simulink model "pump_v000"  (R2019b)
settings: Solver=ode4  StartTime=0.0  StopTime=100  FixedStep=0.02  RelTol=1e-3
libraries: simulink x6
settings Model: PauseTimes=11.82  Creator=engineer  LastModifiedBy=engineer

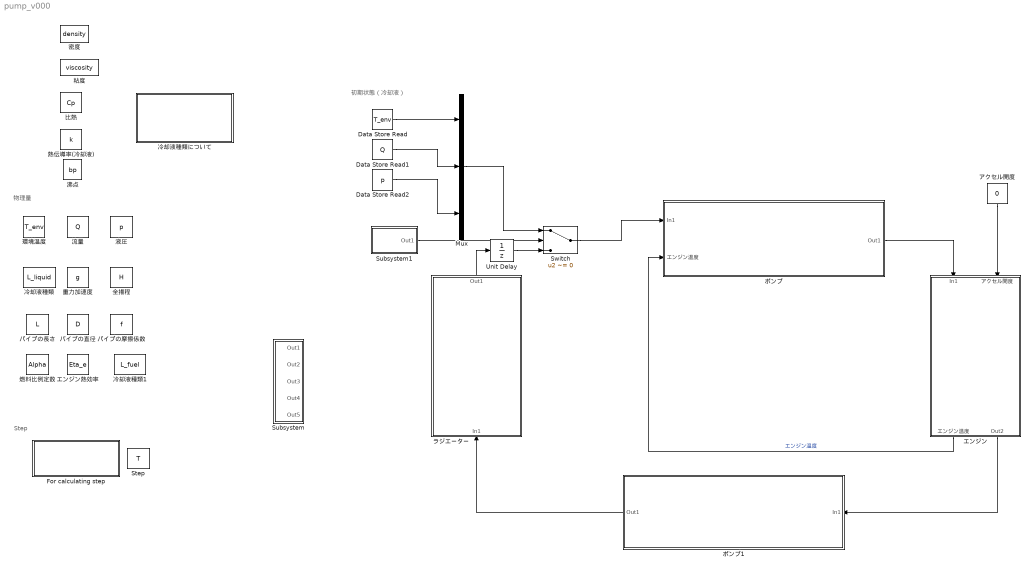
== system pump_v000 ==
  note: 初期状態（冷却液）
  note: 物理量
  note: Step
  " 全揚程" : DataStoreMemory  DataStoreName=H  ReadBeforeWriteMsg=warning  WriteAfterWriteMsg=warning  WriteAfterReadMsg=warning  InitialValue=2  ShowAdditionalParam=off
  " 冷却液種類" : DataStoreMemory  DataStoreName=L_liquid  ReadBeforeWriteMsg=warning  WriteAfterWriteMsg=warning  WriteAfterReadMsg=warning  ShowAdditionalParam=off  OutMin=0  OutMax=2
  " 冷却液種類1" : DataStoreMemory  DataStoreName=L_fuel  ReadBeforeWriteMsg=warning  WriteAfterWriteMsg=warning  WriteAfterReadMsg=warning  ShowAdditionalParam=off  OutMin=0  OutMax=2
  " 流量" : DataStoreMemory  DataStoreName=Q  ReadBeforeWriteMsg=warning  WriteAfterWriteMsg=warning  WriteAfterReadMsg=warning  ShowAdditionalParam=off
  " 液圧" : DataStoreMemory  DataStoreName=p  ReadBeforeWriteMsg=warning  WriteAfterWriteMsg=warning  WriteAfterReadMsg=warning  InitialValue=1  ShowAdditionalParam=off
  " 重力加速度" : DataStoreMemory  DataStoreName=g  ReadBeforeWriteMsg=warning  WriteAfterWriteMsg=warning  WriteAfterReadMsg=warning  InitialValue=10  ShowAdditionalParam=off
  Data Store Read : DataStoreRead  DataStoreName=T_env
  Data Store Read1 : DataStoreRead  DataStoreName=Q
  Data Store Read2 : DataStoreRead  DataStoreName=p
  For calculating step : Subsystem
  Mux : Mux  Inputs=3
  Step : DataStoreMemory  DataStoreName=T  ReadBeforeWriteMsg=warning  WriteAfterWriteMsg=warning  WriteAfterReadMsg=warning  ShowAdditionalParam=off
  Subsystem : Subsystem
  Subsystem1 : Subsystem
  Switch : Switch  Criteria=u2 ~= 0
  Unit Delay : UnitDelay  SampleTime=-1  HasFrameUpgradeWarning=on
  アクセル開度 : Constant  Value=0
  エンジン : Subsystem
  エンジン熱効率 : DataStoreMemory  DataStoreName=Eta_e  ReadBeforeWriteMsg=warning  WriteAfterWriteMsg=warning  WriteAfterReadMsg=warning  InitialValue=0.1  ShowAdditionalParam=off
  パイプの摩擦係数 : DataStoreMemory  DataStoreName=f  ReadBeforeWriteMsg=warning  WriteAfterWriteMsg=warning  WriteAfterReadMsg=warning  InitialValue=0.01  ShowAdditionalParam=off
  パイプの直径 : DataStoreMemory  DataStoreName=D  ReadBeforeWriteMsg=warning  WriteAfterWriteMsg=warning  WriteAfterReadMsg=warning  InitialValue=0.04  ShowAdditionalParam=off
  パイプの長さ : DataStoreMemory  DataStoreName=L  ReadBeforeWriteMsg=warning  WriteAfterWriteMsg=warning  WriteAfterReadMsg=warning  InitialValue=7  ShowAdditionalParam=off
  ポンプ : Subsystem
  ポンプ1 : Subsystem
  ラジエーター : Subsystem
  冷却液種類について : Subsystem
  密度 : DataStoreMemory  DataStoreName=density  ReadBeforeWriteMsg=warning  WriteAfterWriteMsg=warning  WriteAfterReadMsg=warning  ShowAdditionalParam=off
  比熱 : DataStoreMemory  DataStoreName=Cp  ReadBeforeWriteMsg=warning  WriteAfterWriteMsg=warning  WriteAfterReadMsg=warning  ShowAdditionalParam=off
  沸点 : DataStoreMemory  DataStoreName=bp  ReadBeforeWriteMsg=warning  WriteAfterWriteMsg=warning  WriteAfterReadMsg=warning  ShowAdditionalParam=off
  熱伝導率(冷却液) : DataStoreMemory  DataStoreName=k  ReadBeforeWriteMsg=warning  WriteAfterWriteMsg=warning  WriteAfterReadMsg=warning  ShowAdditionalParam=off
  燃料比例定数 : DataStoreMemory  DataStoreName=Alpha  ReadBeforeWriteMsg=warning  WriteAfterWriteMsg=warning  WriteAfterReadMsg=warning  InitialValue=0.005  ShowAdditionalParam=off
  "環境温度 " : DataStoreMemory  DataStoreName=T_env  ReadBeforeWriteMsg=warning  WriteAfterWriteMsg=warning  WriteAfterReadMsg=warning  InitialValue=25  ShowAdditionalParam=off
  粘度 : DataStoreMemory  DataStoreName=viscosity  ReadBeforeWriteMsg=warning  WriteAfterWriteMsg=warning  WriteAfterReadMsg=warning  ShowAdditionalParam=off
  wires:
  ポンプ/1(Out1) -> エンジン/1(In1)
  エンジン/2(Out2) -> ポンプ1/1(In1)
  ポンプ1/1(Out1) -> ラジエーター/1(In1)
  Mux/1 -> Switch/1
  Data Store Read/1 -> Mux/1
  Data Store Read1/1 -> Mux/2
  Data Store Read2/1 -> Mux/3
  Switch/1 -> ポンプ/1(In1)
  ラジエーター/1(Out1) -> Unit Delay/1
  Subsystem1/1(Out1) -> Switch/2
  エンジン/1(エンジン温度) -> ポンプ/2(エンジン温度)  "エンジン温度"
  Unit Delay/1 -> Switch/3
  アクセル開度/1 -> エンジン/2(アクセル開度)

== system pump_v000/For calculating step ==
  Add1 : Sum  Inputs=+-
  Clock1 : Clock
  Data Store Write : DataStoreWrite  DataStoreName=T
  Unit Delay2 : UnitDelay  SampleTime=-1  HasFrameUpgradeWarning=on
  wires:
  Clock1/1 -> Add1/1, Unit Delay2/1
  Add1/1 -> Data Store Write/1
  Unit Delay2/1 -> Add1/2

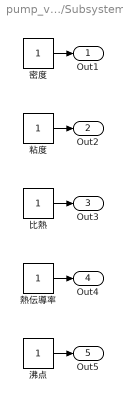
== system pump_v000/Subsystem ==
  密度 : Constant
  比熱 : Constant
  沸点 : Constant
  熱伝導率 : Constant
  粘度 : Constant
  Out1 : Outport
  Out2 : Outport  Port=2
  Out3 : Outport  Port=3
  Out4 : Outport  Port=4
  Out5 : Outport  Port=5
  wires:
  密度/1 -> Out1/1
  沸点/1 -> Out5/1
  比熱/1 -> Out3/1
  粘度/1 -> Out2/1
  熱伝導率/1 -> Out4/1

== system pump_v000/Subsystem1 ==
  Constant : Constant  OutDataTypeStr=boolean
  Logical Operator : Logic  Operator=NOT  AllPortsSameDT=off  OutDataTypeStr=boolean
  Logical Operator1 : Logic  AllPortsSameDT=off  OutDataTypeStr=boolean
  Unit Delay : UnitDelay  SampleTime=-1  HasFrameUpgradeWarning=on
  Out1 : Outport
  wires:
  Constant/1 -> Unit Delay/1, Logical Operator1/1
  Logical Operator/1 -> Logical Operator1/2
  Unit Delay/1 -> Logical Operator/1
  Logical Operator1/1 -> Out1/1

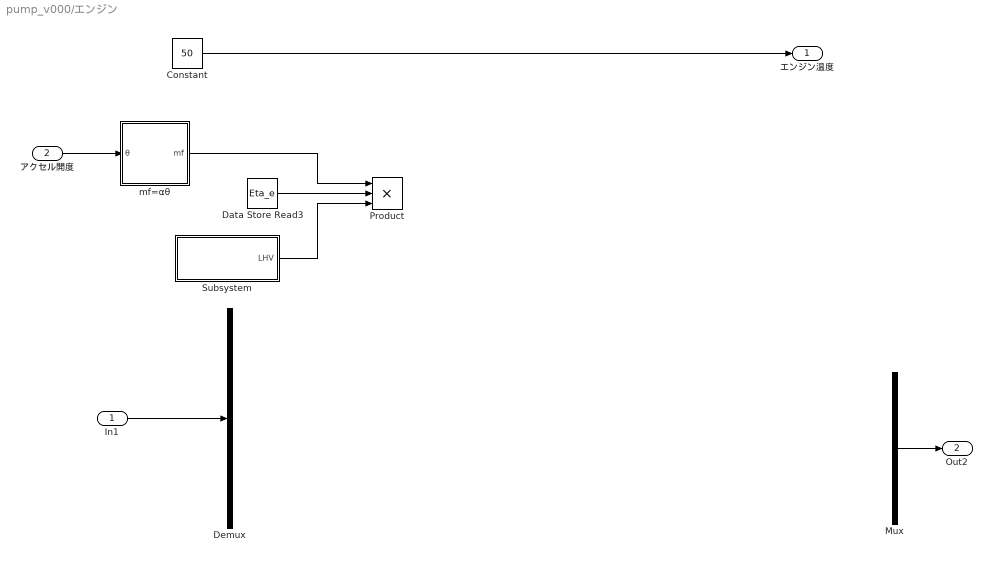
== system pump_v000/エンジン ==
  In1 : Inport
  アクセル開度 : Inport  Port=2
  Constant : Constant  Value=50
  Data Store Read3 : DataStoreRead  DataStoreName=Eta_e
  Demux : Demux  Outputs=3
  Mux : Mux  Inputs=3
  Product : Product  Inputs=3
  Subsystem : Subsystem
  mf=αθ : Subsystem
  エンジン温度 : Outport
  Out2 : Outport  Port=2
  wires:
  In1/1 -> Demux/1
  Constant/1 -> エンジン温度/1
  Mux/1 -> Out2/1
  アクセル開度/1 -> mf=αθ/1(θ)
  mf=αθ/1(mf) -> Product/1
  Data Store Read3/1 -> Product/2
  Subsystem/1("LHV ") -> Product/3

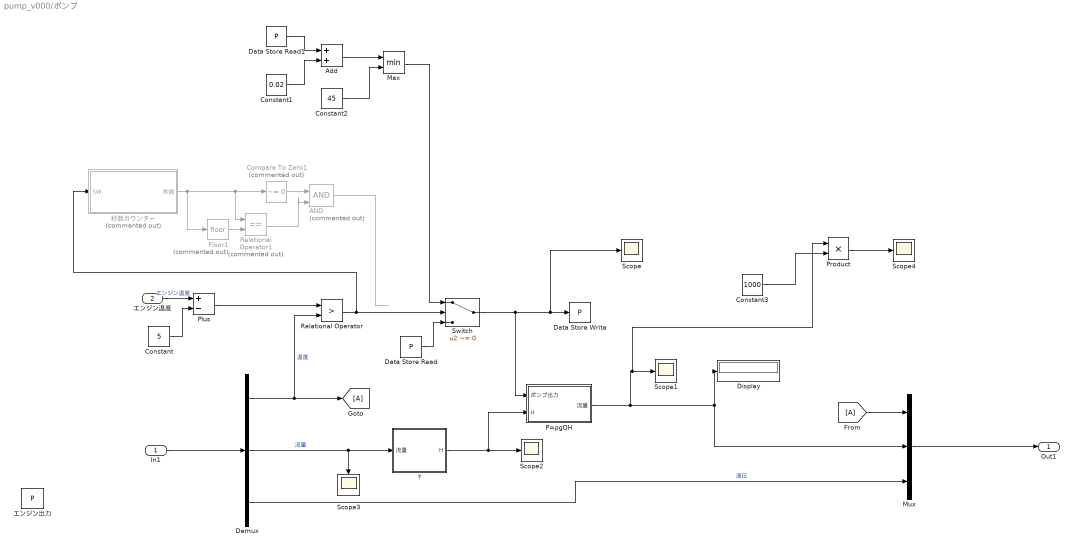
== system pump_v000/ポンプ ==
  In1 : Inport
  エンジン温度 : Inport  Port=2
  "?" : Subsystem
  AND : Logic  Commented=on  IconShape=distinctive  AllPortsSameDT=off  OutDataTypeStr=boolean
  Add : Sum
  Compare To Zero1 : simulink/Logic and Bit Operations/Compare To Zero  Commented=on  relop=~=  OutDataTypeStr=boolean
  Constant : Constant  Value=5
  Constant1 : Constant  Value=0.02
  Constant2 : Constant  Value=45
  Constant3 : Constant  Value=1000
  Data Store Read : DataStoreRead  DataStoreName=P
  Data Store Read1 : DataStoreRead  DataStoreName=P
  Data Store Write : DataStoreWrite  DataStoreName=P
  Demux : Demux  Outputs=3
  Display : Display
  Floor1 : Rounding  Commented=on
  Max : MinMax  Inputs=2
  Mux : Mux  Inputs=3
  P=ρgQH : Subsystem
  Plus : Sum  Inputs=+-
  Product : Product
  Relational Operator : RelationalOperator  Operator=>  OutDataTypeStr=boolean  RndMeth=Simplest
  Relational Operator1 : RelationalOperator  Commented=on  Operator===  OutDataTypeStr=boolean  RndMeth=Simplest
  Scope{,1..4} (5 alike) : Scope
  Switch : Switch  Criteria=u2 ~= 0
  エンジン出力 : DataStoreMemory  DataStoreName=P  ReadBeforeWriteMsg=warning  WriteAfterWriteMsg=warning  WriteAfterReadMsg=warning  ShowAdditionalParam=off
  秒数カウンター : Subsystem  Commented=on
  Out1 : Outport
  wires:
  In1/1 -> Demux/1
  Demux/3 -> Mux/3  "液圧"
  Demux/1 -> Relational Operator/2, [A]  "温度"
  P=ρgQH/1(流量) -> Display/1, Mux/2, Product/1, Scope1/1
  Constant/1 -> Plus/2
  エンジン温度/1 -> Plus/1  "エンジン温度"
  Plus/1 -> Relational Operator/1
  Switch/1 -> P=ρgQH/1(ポンプ出力), Scope/1, Data Store Write/1
  Data Store Read/1 -> Switch/3
  Data Store Read1/1 -> Add/1
  Constant1/1 -> Add/2
  Constant2/1 -> Max/2
  Add/1 -> Max/1
  Mux/1 -> Out1/1
  Demux/2 -> "?"/1(流量), Scope3/1  "流量"
  "?"/1(H) -> Scope2/1, P=ρgQH/2(H)
  [A] -> Mux/1
  Relational Operator1/1 -> AND/2
  秒数カウンター/1(秒数) -> Compare To Zero1/1, Relational Operator1/1, Floor1/1
  Floor1/1 -> Relational Operator1/2
  Compare To Zero1/1 -> AND/1
  AND/1 -> ?
  Max/1 -> Switch/1
  Relational Operator/1 -> Switch/2, 秒数カウンター/1(SW)
  Constant3/1 -> Product/2
  Product/1 -> Scope4/1

== system pump_v000/ポンプ1 ==
  In1 : Inport
  Out1 : Outport
  wires:
  In1/1 -> Out1/1

== system pump_v000/ラジエーター ==
  In1 : Inport
  Out1 : Outport
  wires:
  In1/1 -> Out1/1

== system pump_v000/冷却液種類について ==
  Compare To Constant : simulink/Logic and Bit Operations/Compare To Constant  relop===  const=0  OutDataTypeStr=boolean
  Compare To Constant1 : simulink/Logic and Bit Operations/Compare To Constant  relop===  const=1  OutDataTypeStr=boolean
  Compare To Constant2 : simulink/Logic and Bit Operations/Compare To Constant  relop===  const=2  OutDataTypeStr=boolean
  Data Store Read3 : DataStoreRead  DataStoreName=L_liquid
  Enabled Subsystem : Subsystem  TreatAsAtomicUnit=on
  Enabled Subsystem1 : Subsystem  TreatAsAtomicUnit=on
  Enabled Subsystem3 : Subsystem  TreatAsAtomicUnit=on
  wires:
  Compare To Constant/1 -> Enabled Subsystem/Enable  "水"
  Data Store Read3/1 -> Compare To Constant2/1, Compare To Constant1/1, Compare To Constant/1
  Compare To Constant1/1 -> Enabled Subsystem3/Enable  "EG(30%)"
  Compare To Constant2/1 -> Enabled Subsystem1/Enable  "EG(50%)"

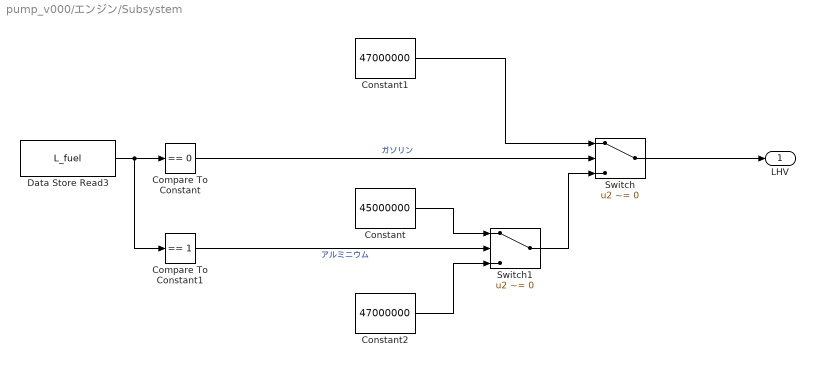
== system pump_v000/エンジン/Subsystem ==
  Compare To Constant : simulink/Logic and Bit Operations/Compare To Constant  relop===  const=0  OutDataTypeStr=boolean
  Compare To Constant1 : simulink/Logic and Bit Operations/Compare To Constant  relop===  const=1  OutDataTypeStr=boolean
  Constant : Constant  Value=45000000
  Constant1 : Constant  Value=47000000
  Constant2 : Constant  Value=47000000
  Data Store Read3 : DataStoreRead  DataStoreName=L_fuel
  Switch : Switch  Criteria=u2 ~= 0
  Switch1 : Switch  Criteria=u2 ~= 0
  "LHV " : Outport
  wires:
  Compare To Constant1/1 -> Switch1/2  "アルミニウム"
  Data Store Read3/1 -> Compare To Constant1/1, Compare To Constant/1
  Compare To Constant/1 -> Switch/2  "ガソリン"
  Switch/1 -> "LHV "/1
  Constant1/1 -> Switch/1
  Switch1/1 -> Switch/3
  Constant/1 -> Switch1/1
  Constant2/1 -> Switch1/3

== system pump_v000/エンジン/mf=αθ ==
  θ : Inport
  Constant1 : Constant  Value=0.02
  Data Store Read3 : DataStoreRead  DataStoreName=Alpha
  Product : Product  Inputs=3
  mf : Outport
  wires:
  Product/1 -> mf/1
  Data Store Read3/1 -> Product/2
  Constant1/1 -> Product/3
  θ/1 -> Product/1

== system pump_v000/ポンプ/? ==
  note: ?
  流量 : Inport
  Scope : Scope
  Scope1 : Scope
  hf=(fLv^2)/(2gD) : Subsystem
  v=Q/A : Subsystem
  ベルヌーイの定理 : Subsystem
  H : Outport
  wires:
  流量/1 -> Scope1/1, v=Q/A/1(Q)
  hf=(fLv^2)/(2gD)/1(hf) -> ベルヌーイの定理/1(hf)
  v=Q/A/1(v) -> ベルヌーイの定理/2(v), hf=(fLv^2)/(2gD)/1(v)
  ベルヌーイの定理/1(H) -> Scope/1, H/1

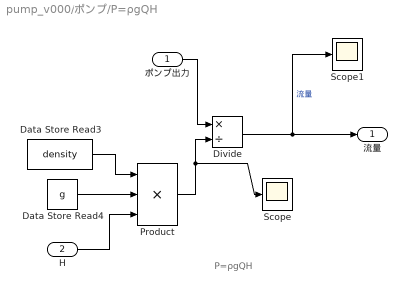
== system pump_v000/ポンプ/P=ρgQH ==
  note: P=ρgQH
  ポンプ出力 : Inport
  H : Inport  Port=2
  Data Store Read3 : DataStoreRead  DataStoreName=density
  Data Store Read4 : DataStoreRead  DataStoreName=g
  Divide : Product  Inputs=*/
  Product : Product  Inputs=3
  Scope : Scope
  Scope1 : Scope
  流量 : Outport
  wires:
  H/1 -> Product/3
  Data Store Read3/1 -> Product/1
  ポンプ出力/1 -> Divide/1
  Data Store Read4/1 -> Product/2
  Product/1 -> Scope/1, Divide/2
  Divide/1 -> Scope1/1, 流量/1  "流量"

== system pump_v000/ポンプ/秒数カウンター ==
  SW : Inport
  Add : Sum
  Constant1 : Constant  Value=0
  Data Store Read : DataStoreRead  DataStoreName=T
  Switch2 : Switch  Criteria=u2 ~= 0
  Unit Delay1 : UnitDelay  SampleTime=-1  HasFrameUpgradeWarning=on
  秒数 : Outport
  wires:
  SW/1 -> Switch2/2
  Add/1 -> Switch2/1
  Data Store Read/1 -> Add/2
  Constant1/1 -> Switch2/3
  Switch2/1 -> 秒数/1, Unit Delay1/1
  Unit Delay1/1 -> Add/1

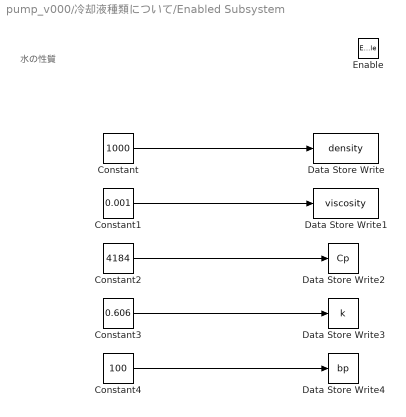
== system pump_v000/冷却液種類について/Enabled Subsystem ==
  note: 水の性質
  Enable : EnablePort
  Constant : Constant  Value=1000
  Constant1 : Constant  Value=0.001
  Constant2 : Constant  Value=4184
  Constant3 : Constant  Value=0.606
  Constant4 : Constant  Value=100
  Data Store Write : DataStoreWrite  DataStoreName=density
  Data Store Write1 : DataStoreWrite  DataStoreName=viscosity
  Data Store Write2 : DataStoreWrite  DataStoreName=Cp
  Data Store Write3 : DataStoreWrite  DataStoreName=k
  Data Store Write4 : DataStoreWrite  DataStoreName=bp
  wires:
  Constant/1 -> Data Store Write/1
  Constant1/1 -> Data Store Write1/1
  Constant2/1 -> Data Store Write2/1
  Constant3/1 -> Data Store Write3/1
  Constant4/1 -> Data Store Write4/1

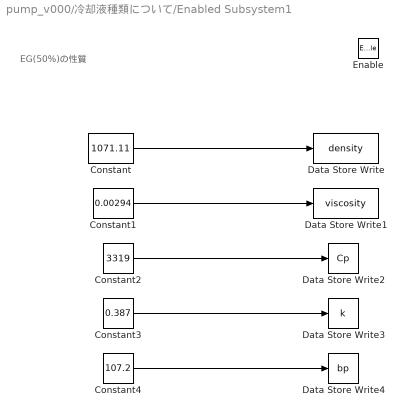
== system pump_v000/冷却液種類について/Enabled Subsystem1 ==
  note: EG(50%)の性質
  Enable : EnablePort
  Constant : Constant  Value=1071.11
  Constant1 : Constant  Value=0.00294
  Constant2 : Constant  Value=3319
  Constant3 : Constant  Value=0.387
  Constant4 : Constant  Value=107.2
  Data Store Write : DataStoreWrite  DataStoreName=density
  Data Store Write1 : DataStoreWrite  DataStoreName=viscosity
  Data Store Write2 : DataStoreWrite  DataStoreName=Cp
  Data Store Write3 : DataStoreWrite  DataStoreName=k
  Data Store Write4 : DataStoreWrite  DataStoreName=bp
  wires:
  Constant/1 -> Data Store Write/1
  Constant1/1 -> Data Store Write1/1
  Constant2/1 -> Data Store Write2/1
  Constant3/1 -> Data Store Write3/1
  Constant4/1 -> Data Store Write4/1

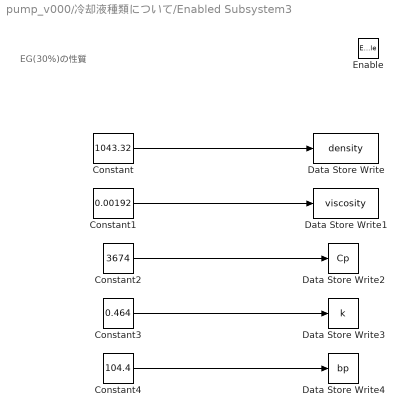
== system pump_v000/冷却液種類について/Enabled Subsystem3 ==
  note: EG(30%)の性質
  Enable : EnablePort
  Constant : Constant  Value=1043.32
  Constant1 : Constant  Value=0.00192
  Constant2 : Constant  Value=3674
  Constant3 : Constant  Value=0.464
  Constant4 : Constant  Value=104.4
  Data Store Write : DataStoreWrite  DataStoreName=density
  Data Store Write1 : DataStoreWrite  DataStoreName=viscosity
  Data Store Write2 : DataStoreWrite  DataStoreName=Cp
  Data Store Write3 : DataStoreWrite  DataStoreName=k
  Data Store Write4 : DataStoreWrite  DataStoreName=bp
  wires:
  Constant/1 -> Data Store Write/1
  Constant1/1 -> Data Store Write1/1
  Constant2/1 -> Data Store Write2/1
  Constant3/1 -> Data Store Write3/1
  Constant4/1 -> Data Store Write4/1

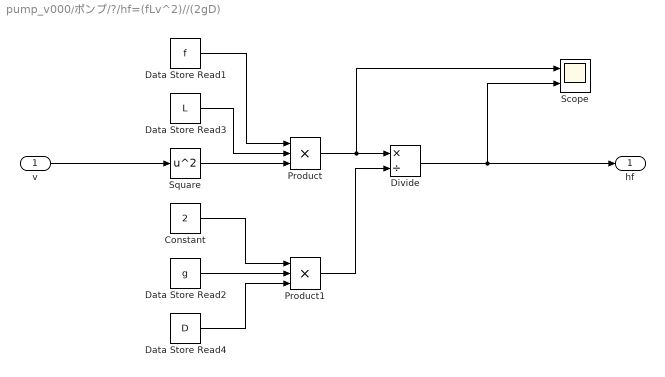
== system pump_v000/ポンプ/?/hf=(fLv^2)//(2gD) ==
  v : Inport
  Constant : Constant  Value=2
  Data Store Read1 : DataStoreRead  DataStoreName=f
  Data Store Read2 : DataStoreRead  DataStoreName=g
  Data Store Read3 : DataStoreRead  DataStoreName=L
  Data Store Read4 : DataStoreRead  DataStoreName=D
  Divide : Product  Inputs=*/
  Product : Product  Inputs=3
  Product1 : Product  Inputs=3
  Scope : Scope  NumInputPorts=2
  Square : Math  Operator=square  SignedPower=off  SaturateOnIntegerOverflow=on
  hf : Outport
  wires:
  v/1 -> Square/1
  Square/1 -> Product/3
  Data Store Read3/1 -> Product/2
  Data Store Read1/1 -> Product/1
  Product/1 -> Scope/1, Divide/1
  Constant/1 -> Product1/1
  Data Store Read2/1 -> Product1/2
  Data Store Read4/1 -> Product1/3
  Product1/1 -> Divide/2
  Divide/1 -> Scope/2, hf/1

== system pump_v000/ポンプ/?/v=Q//A ==
  Q : Inport
  A=pi*(D/2)^2 : Subsystem
  Divide1 : Product  Inputs=*/
  v : Outport
  wires:
  Q/1 -> Divide1/1
  Divide1/1 -> v/1
  A=pi*(D/2)^2/1(A) -> Divide1/2

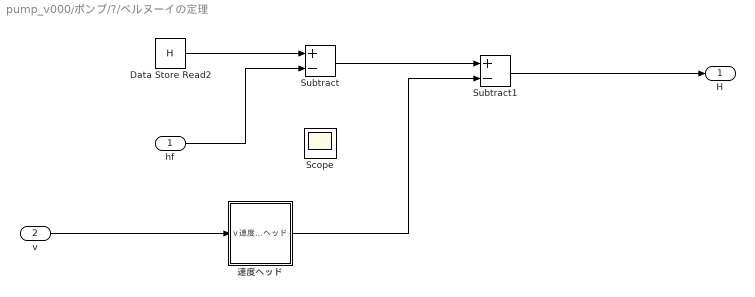
== system pump_v000/ポンプ/?/ベルヌーイの定理 ==
  hf : Inport
  v : Inport  Port=2
  Data Store Read2 : DataStoreRead  DataStoreName=H
  Scope : Scope
  Subtract : Sum  Inputs=+-
  Subtract1 : Sum  Inputs=+-
  速度ヘッド : Subsystem
  H : Outport
  wires:
  Data Store Read2/1 -> Subtract/1
  Subtract/1 -> Subtract1/1
  v/1 -> 速度ヘッド/1(v)
  速度ヘッド/1(速度ヘッド) -> Subtract1/2
  hf/1 -> Subtract/2
  Subtract1/1 -> H/1

== system pump_v000/ポンプ/?/v=Q//A/A=pi*(D//2)^2 ==
  Constant : Constant  Value=2
  Data Store Read3 : DataStoreRead  DataStoreName=D
  Divide : Product  Inputs=*/
  Pi : Constant  Value=pi  OutDataTypeStr=Inherit: Inherit via back propagation
  Product : Product
  Square : Math  Operator=square  SignedPower=off  SaturateOnIntegerOverflow=on
  A : Outport
  wires:
  Constant/1 -> Divide/2
  Divide/1 -> Square/1
  Data Store Read3/1 -> Divide/1
  Product/1 -> A/1
  Pi/1 -> Product/2
  Square/1 -> Product/1

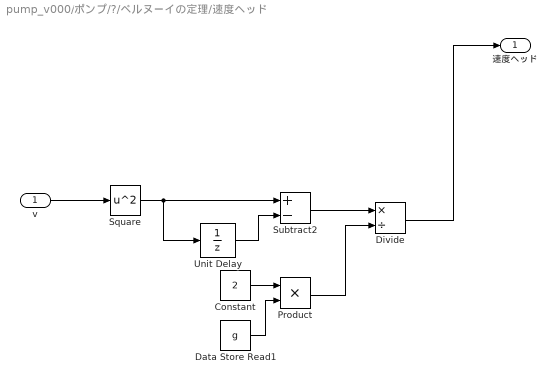
== system pump_v000/ポンプ/?/ベルヌーイの定理/速度ヘッド ==
  v : Inport
  Constant : Constant  Value=2
  Data Store Read1 : DataStoreRead  DataStoreName=g
  Divide : Product  Inputs=*/
  Product : Product
  Square : Math  Operator=square  SignedPower=off  SaturateOnIntegerOverflow=on
  Subtract2 : Sum  Inputs=+-
  Unit Delay : UnitDelay  SampleTime=-1  HasFrameUpgradeWarning=on
  速度ヘッド : Outport
  wires:
  Constant/1 -> Product/1
  v/1 -> Square/1
  Product/1 -> Divide/2
  Unit Delay/1 -> Subtract2/2
  Square/1 -> Unit Delay/1, Subtract2/1
  Data Store Read1/1 -> Product/2
  Divide/1 -> 速度ヘッド/1
  Subtract2/1 -> Divide/1
